simulink model "angular_acceleration"  (Simulink 7.1)
settings: Solver=ode45  StartTime=0.0  StopTime=10.0  RelTol=1e-3
settings Model: Creator=s0237326  LastModifiedBy=s0237326

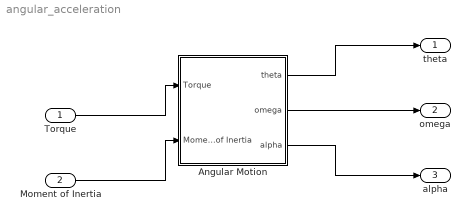
== system angular_acceleration ==
  Torque : Inport  OutDataType=sfix(16)  OutScaling=2^0
  Moment of Inertia : Inport  Port=2  OutDataType=sfix(16)  OutScaling=2^0
  Angular Motion : Subsystem
  theta : Outport  OutDataType=sfix(16)  OutScaling=2^0
  omega : Outport  Port=2  OutDataType=sfix(16)  OutScaling=2^0
  alpha : Outport  Port=3  OutDataType=sfix(16)  OutScaling=2^0
  wires:
  Angular Motion/1(theta) -> theta/1
  Angular Motion/2(omega) -> omega/1
  Torque/1 -> Angular Motion/1(Torque)
  Angular Motion/3(alpha) -> alpha/1
  Moment of Inertia/1 -> Angular Motion/2(Moment of Inertia)

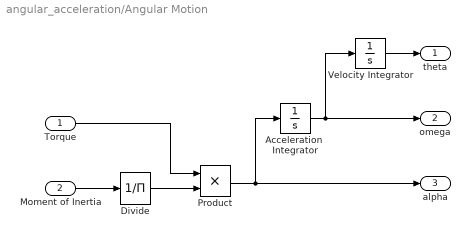
== system angular_acceleration/Angular Motion ==
  Torque : Inport  OutDataType=sfix(16)  OutScaling=2^0
  Moment of Inertia : Inport  Port=2  OutDataType=sfix(16)  OutScaling=2^0
  Acceleration  Integrator : Integrator
  Divide : Product  Inputs=/  OutDataType=sfix(16)  OutScaling=2^-10
  Product : Product  OutDataType=sfix(16)  OutScaling=2^0  RndMeth=Zero
  Velocity Integrator : Integrator
  theta : Outport  OutDataType=sfix(16)  OutScaling=2^0
  omega : Outport  Port=2  OutDataType=sfix(16)  OutScaling=2^0
  alpha : Outport  Port=3  OutDataType=sfix(16)  OutScaling=2^0
  wires:
  Product/1 -> alpha/1, Acceleration  Integrator/1
  Velocity Integrator/1 -> theta/1
  Acceleration  Integrator/1 -> omega/1, Velocity Integrator/1
  Torque/1 -> Product/1
  Moment of Inertia/1 -> Divide/1
  Divide/1 -> Product/2
